simulink library "ASDRouter"  (R2022b)
settings: Solver=VariableStepAuto  StartTime=0.0  StopTime=10.0  RelTol=1e-3
undefined symbols (not defined in the file or in its folder): aux_gain, enable_aux, L, main_gain, main_select, num_aux_chs, num_main_chs, num_output_chs
libraries: simulink x2, AsdRouterBtc x1, dspindex x1
settings Model: Creator=darshana.mistry  LastModifiedBy=kl13806
settings SolverCC: AlgebraicLoopSolver=TrustRegion
settings DebuggingCC: UnconnectedInputMsg=warning  UnconnectedOutputMsg=warning  UnconnectedLineMsg=warning  SFMachineParentedDataDiag=warning  ArithmeticOperatorsInVariantConditions=warning
settings ModelReferenceCC: EnableRefExpFcnMdlSchedulingChecks=on
settings SFSimCC: CustomCodeUndefinedFunction=UseInterfaceOnly
settings RTWCC: DLArmComputeVersion=19.05

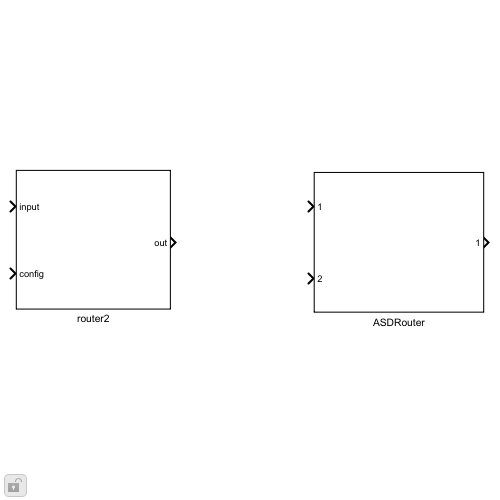
[thumbnail: Simulink's stored preview of the top-level diagram]
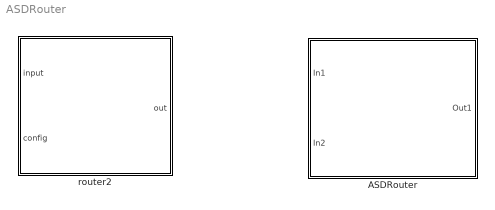
== system ASDRouter ==
  ASDRouter : Subsystem  mask{frameSize=L, nChanOut=num_output_chs, mainSelect=main_select, numMainCh=num_main_chs, mainGain=main_gain, enableAux=enable_aux, numAux=num_aux_chs, auxGain=aux_gain}
      mask prompts: frameSize "Frame Size (L)"; nChanOut "Number of Output Channels"; mainSelect "Main Channel Select Vector"; numMainCh "Number of Main Channels"; mainGain "Main gain for each output channel"; enableAux "Enable Aux input sources"; numAux "Number of Aux Channels"; auxGain "Aux gain for each output channel for each Aux source"
      mask init:
      | blkh = gcbh;
      | % Copy discrete mask parameters into a classdef object
      | InnerLinkConfig = AsdRouterConfig;
      | InnerLinkConfig.FrameSize = frameSize;
      | InnerLinkConfig.NumChanOut = nChanOut;
      | InnerLinkConfig.MainSelect = mainSelect;
      | InnerLinkConfig.NumMainCh = numMainCh;
      | InnerLinkConfig.MainGain = mainGain;
      | InnerLinkConfig.EnableAux = enableAux;
      | InnerLinkConfig.NumAux = numAux;
      | InnerLinkConfig.AuxGain = auxGain;
  router2 : Subsystem  mask{router_input_length=4}

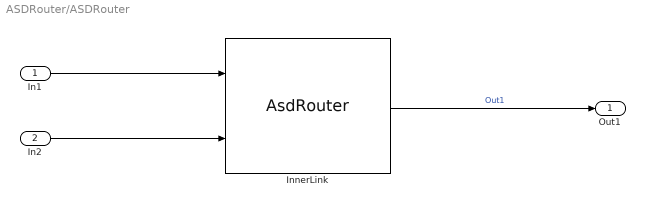
== system ASDRouter/ASDRouter ==
  In1 : Inport
  In2 : Inport  Port=2
  InnerLink : AsdRouterBtc/AsdRouter  Config=InnerLinkConfig  FeatureName=ASDRouter
      settings: SourceProductName=Bose Blocklib
  Out1 : Outport
  wires:
  InnerLink/1 -> Out1/1  "Out1"
  In1/1 -> InnerLink/1
  In2/1 -> InnerLink/2

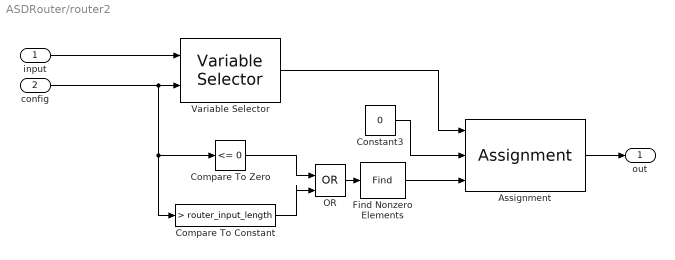
== system ASDRouter/router2 ==
  input : Inport
  config : Inport  Port=2
  Assignment : Assignment  NumberOfDimensions=2  DiagnosticForDimensions=Warning  IndexOptions=Assign all,Index vector (port)  Indices=1,[1 3]  OutputSizes=1,1
  Compare To Constant : simulink/Logic and Bit Operations/Compare To Constant  relop=>  const=router_input_length  OutDataTypeStr=boolean
  Compare To Zero : simulink/Logic and Bit Operations/Compare To Zero  relop=<=  OutDataTypeStr=boolean
  Constant3 : Constant  Value=0  OutDataTypeStr=single
  Find Nonzero Elements : Find  NumberOfInputDimensions=3
  OR : Logic  Operator=OR  IconShape=distinctive  AllPortsSameDT=off  OutDataTypeStr=boolean
  Variable Selector : dspindex/Variable Selector  NumInputs=1  rowsOrCols=Columns  IdxMode=Variable  Elements=[3]  ZerOneIdxMode=One-based  errmode=Clip Index  FillMode=on  FillValues=0
  out : Outport  VectorParamsAs1DForOutWhenUnconnected=off
  wires:
  Compare To Constant/1 -> OR/2
  Assignment/1 -> out/1
  OR/1 -> Find Nonzero Elements/1
  config/1 -> Compare To Constant/1, Compare To Zero/1, Variable Selector/2
  Variable Selector/1 -> Assignment/1
  Find Nonzero Elements/1 -> Assignment/3
  input/1 -> Variable Selector/1
  Compare To Zero/1 -> OR/1
  Constant3/1 -> Assignment/2
